simulink model "testBode"  (R2020b)
settings: Solver=VariableStepAuto  StartTime=0.0  StopTime=10.0  RelTol=1e-3
settings Model: Creator=kaijunge  LastModifiedBy=kaijunge

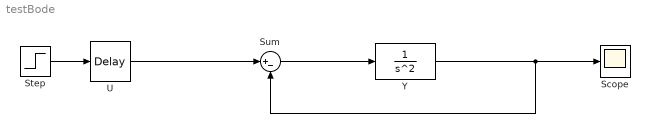
== system testBode ==
  Scope : Scope
  Step : Step  SampleTime=0
  Sum : Sum  Inputs=|+-
  U : TransportDelay
  Y : TransferFcn  Denominator=[1 0 0]
  wires:
  Y/1 -> Sum/2, Scope/1
  Sum/1 -> Y/1
  Step/1 -> U/1
  U/1 -> Sum/1
